simulink model "scope_model_lab_1"  (R2021b)
settings: Solver=VariableStepAuto  StartTime=0.0  StopTime=1  MaxStep=1e-3  RelTol=1e-3
values from neighbouring files (symbols this model uses):
  a11 = -3    [script_lab_1.m]
  a12 = -2    [script_lab_1.m]
  a21 = -5    [script_lab_1.m]
  a22 = -6    [script_lab_1.m]
  b11 = 3    [script_lab_1.m]
  b12 = 7    [script_lab_1.m]
settings Model: Creator=79159  LastModifiedBy=79159

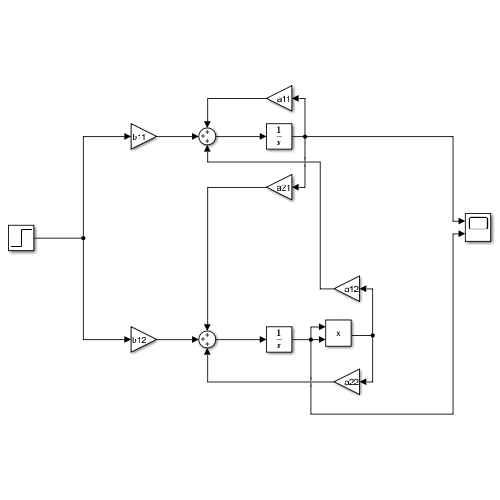
[thumbnail: Simulink's stored preview of the top-level diagram]
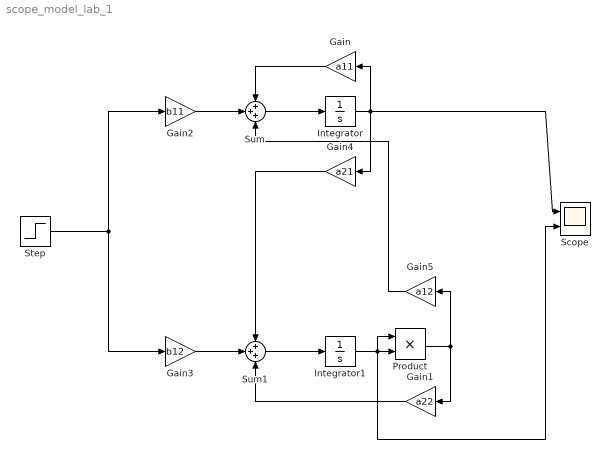
== system scope_model_lab_1 ==
  Gain : Gain  Gain=a11
  Gain1 : Gain  Gain=a22
  Gain2 : Gain  Gain=b11
  Gain3 : Gain  Gain=b12
  Gain4 : Gain  Gain=a21
  Gain5 : Gain  Gain=a12
  Integrator : Integrator
  Integrator1 : Integrator
  Product : Product
  Scope : Scope  NumInputPorts=2
  Step : Step  Time=0  After=u  SampleTime=0
  Sum : Sum  Inputs=+++
  Sum1 : Sum  Inputs=+++
  wires:
  Integrator/1 -> Gain4/1, Scope/1, Gain/1
  Sum1/1 -> Integrator1/1
  Sum/1 -> Integrator/1
  Gain3/1 -> Sum1/2
  Gain2/1 -> Sum/2
  Step/1 -> Gain2/1, Gain3/1
  Gain/1 -> Sum/1
  Gain4/1 -> Sum1/1
  Gain1/1 -> Sum1/3
  Gain5/1 -> Sum/3
  Integrator1/1 -> Product/1, Scope/2, Product/2
  Product/1 -> Gain5/1, Gain1/1
